simulink model "corrsys"  (R2021a)
settings: Solver=VariableStepAuto  StartTime=0.0  StopTime=0.5  RelTol=1e-3
libraries: slctrlblks x7
settings Model: Creator=Евгений  LastModifiedBy=Евгений

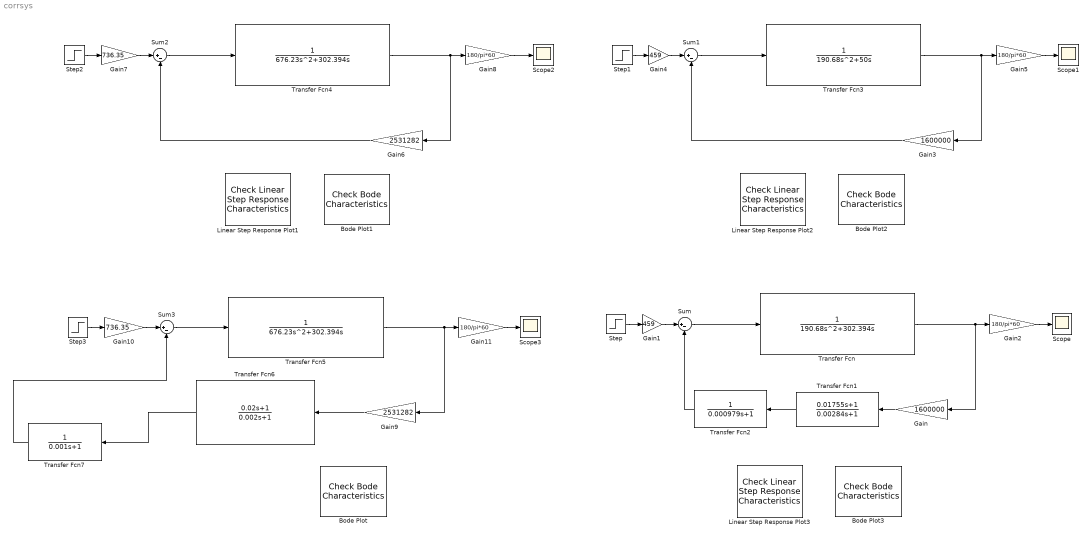
== system corrsys ==
  Bode Plot : slctrlblks/Model Verification/Check Bode  Characteristics  InstantiateOnLoad=on  SaveOperatingPoints=off  LinearizationIOs={'/Gain10', 1, 'in', 'off', '';'/Transfer Fcn7', 1, 'out', 'on', ''}  LinearizeAt=SnapshotTimes  SnapshotTimes=[0]  TriggerType=rising  SampleTime=auto  RateConversionMethod=zoh  PreWarpFreq=10  UseExactDelayModel=off  UseFullBlockNameLabels=off  UseBusSignalLabels=off  enabled=on  stopWhenAssertionFail=off  export=off  ViewDlgPos=[4 4 449 431]  OpenViewOnLoad=off  LaunchViewOnOpen=off  FrequencyUnits=rad/s  MagnitudeUnits=dB  PhaseUnits=deg  TimeUnits=seconds  EnableUpperBound=off  UpperBoundFrequencies=[]  UpperBoundMagnitudes=[]  EnableLowerBound=on  LowerBoundFrequencies=[]  LowerBoundMagnitudes=[]
  Bode Plot1 : slctrlblks/Model Verification/Check Bode  Characteristics  InstantiateOnLoad=on  SaveOperatingPoints=off  LinearizationIOs={'/Gain7', 1, 'in', 'off', '';'/Gain6', 1, 'out', 'on', ''}  LinearizeAt=SnapshotTimes  SnapshotTimes=[0]  TriggerType=rising  SampleTime=auto  RateConversionMethod=zoh  PreWarpFreq=10  UseExactDelayModel=off  UseFullBlockNameLabels=off  UseBusSignalLabels=off  enabled=on  stopWhenAssertionFail=off  export=off  ViewDlgPos=[1 1 1826 895]  OpenViewOnLoad=on  LaunchViewOnOpen=off  FrequencyUnits=rad/s  MagnitudeUnits=dB  PhaseUnits=deg  TimeUnits=seconds  EnableUpperBound=off  UpperBoundFrequencies=[]  UpperBoundMagnitudes=[]  EnableLowerBound=on  LowerBoundFrequencies=[]  LowerBoundMagnitudes=[]
  Bode Plot2 : slctrlblks/Model Verification/Check Bode  Characteristics  InstantiateOnLoad=on  SaveOperatingPoints=off  LinearizationIOs={'/Gain4', 1, 'in', 'off', '';'/Gain3', 1, 'out', 'on', ''}  LinearizeAt=SnapshotTimes  SnapshotTimes=[0]  TriggerType=rising  SampleTime=auto  RateConversionMethod=zoh  PreWarpFreq=10  UseExactDelayModel=off  UseFullBlockNameLabels=off  UseBusSignalLabels=off  enabled=on  stopWhenAssertionFail=off  export=off  ViewDlgPos=[100 200 510 390]  OpenViewOnLoad=off  LaunchViewOnOpen=off  FrequencyUnits=rad/s  MagnitudeUnits=dB  PhaseUnits=deg  TimeUnits=seconds  EnableUpperBound=off  UpperBoundFrequencies=[]  UpperBoundMagnitudes=[]  EnableLowerBound=off  LowerBoundFrequencies=[]  LowerBoundMagnitudes=[]
  Bode Plot3 : slctrlblks/Model Verification/Check Bode  Characteristics  InstantiateOnLoad=on  SaveOperatingPoints=off  LinearizationIOs={'/Gain1', 1, 'in', 'off', '';'/Transfer Fcn2', 1, 'out', 'on', ''}  LinearizeAt=SnapshotTimes  SnapshotTimes=[0]  TriggerType=rising  SampleTime=auto  RateConversionMethod=zoh  PreWarpFreq=10  UseExactDelayModel=off  UseFullBlockNameLabels=off  UseBusSignalLabels=off  enabled=on  stopWhenAssertionFail=off  export=off  ViewDlgPos=[4 5 573 384]  OpenViewOnLoad=off  LaunchViewOnOpen=off  FrequencyUnits=rad/s  MagnitudeUnits=dB  PhaseUnits=deg  TimeUnits=seconds  EnableUpperBound=off  UpperBoundFrequencies=[]  UpperBoundMagnitudes=[]  EnableLowerBound=on  LowerBoundFrequencies=[]  LowerBoundMagnitudes=[]
  Gain : Gain  Gain=1600000
  Gain1 : Gain  Gain=459
  Gain10 : Gain  Gain=736.35
  Gain{2,5,8,11} (4 alike) : Gain  Gain=180/pi*60
  Gain3 : Gain  Gain=1600000
  Gain4 : Gain  Gain=459
  Gain6 : Gain  Gain=2531282
  Gain7 : Gain  Gain=736.35
  Gain9 : Gain  Gain=2531282
  Linear Step Response Plot1 : slctrlblks/Model Verification/Check Linear Step Response Characteristics  InstantiateOnLoad=on  SaveOperatingPoints=off  LinearizationIOs={'/Step2', 1, 'in', 'off', '';'/Gain8', 1, 'out', 'off', ''}  LinearizeAt=SnapshotTimes  SnapshotTimes=[0]  TriggerType=rising  SampleTime=auto  RateConversionMethod=zoh  PreWarpFreq=10  UseExactDelayModel=off  UseFullBlockNameLabels=off  UseBusSignalLabels=off  enabled=on  stopWhenAssertionFail=off  export=off  ViewDlgPos=[1372 4 449 431]  OpenViewOnLoad=off  LaunchViewOnOpen=off  FrequencyUnits=rad/s  MagnitudeUnits=dB  PhaseUnits=deg  TimeUnits=seconds  EnableStepResponseBound=off  FinalValue=[]  RiseTime=[]  PercentRise=[]  SettlingTime=[]  PercentSettling=[]  PercentOvershoot=[]  PercentUndershoot=[]
      settings: SourceProductBaseCode=SD  SaveToWorkspace=off  SaveName=sys
  Linear Step Response Plot2 : slctrlblks/Model Verification/Check Linear Step Response Characteristics  InstantiateOnLoad=on  SaveOperatingPoints=off  LinearizationIOs={'/Step1', 1, 'in', 'off', '';'/Gain5', 1, 'out', 'off', ''}  LinearizeAt=SnapshotTimes  SnapshotTimes=[0]  TriggerType=rising  SampleTime=auto  RateConversionMethod=zoh  PreWarpFreq=10  UseExactDelayModel=off  UseFullBlockNameLabels=off  UseBusSignalLabels=off  enabled=on  stopWhenAssertionFail=off  export=off  ViewDlgPos=[584 417 573 384]  OpenViewOnLoad=off  LaunchViewOnOpen=off  FrequencyUnits=rad/s  MagnitudeUnits=dB  PhaseUnits=deg  TimeUnits=seconds  EnableStepResponseBound=off  FinalValue=[]  RiseTime=[]  PercentRise=[]  SettlingTime=[]  PercentSettling=[]  PercentOvershoot=[]  PercentUndershoot=[]
      settings: SourceProductBaseCode=SD  SaveToWorkspace=off  SaveName=sys
  Linear Step Response Plot3 : slctrlblks/Model Verification/Check Linear Step Response Characteristics  InstantiateOnLoad=on  SaveOperatingPoints=off  LinearizationIOs={'/Step', 1, 'in', 'off', '';'/Gain2', 1, 'out', 'off', ''}  LinearizeAt=SnapshotTimes  SnapshotTimes=[0]  TriggerType=rising  SampleTime=auto  RateConversionMethod=zoh  PreWarpFreq=10  UseExactDelayModel=off  UseFullBlockNameLabels=off  UseBusSignalLabels=off  enabled=on  stopWhenAssertionFail=off  export=off  ViewDlgPos=[584 5 573 384]  OpenViewOnLoad=off  LaunchViewOnOpen=off  FrequencyUnits=rad/s  MagnitudeUnits=dB  PhaseUnits=deg  TimeUnits=seconds  EnableStepResponseBound=off  FinalValue=[]  RiseTime=[]  PercentRise=[]  SettlingTime=[]  PercentSettling=[]  PercentOvershoot=[]  PercentUndershoot=[]
      settings: SourceProductBaseCode=SD  SaveToWorkspace=off  SaveName=sys
  Scope{,1..3} (4 alike) : Scope
  Step{,1..3} (4 alike) : Step  Time=0  SampleTime=0
  Sum{,1..3} (4 alike) : Sum  Inputs=|+-
  Transfer Fcn : TransferFcn  Denominator=[190.68 302.394 0]
  Transfer Fcn1 : TransferFcn  Numerator="[0.01755  1]"  Denominator=[0.00284 1]
  Transfer Fcn2 : TransferFcn  Denominator=[0.000979 1]
  Transfer Fcn3 : TransferFcn  Denominator=[190.68 50 0]
  Transfer Fcn4 : TransferFcn  Denominator=[676.23 302.394 0]
  Transfer Fcn5 : TransferFcn  Denominator=[676.23 302.394 0]
  Transfer Fcn6 : TransferFcn  Numerator=[0.02 1]  Denominator=[0.002 1]
  Transfer Fcn7 : TransferFcn  Denominator="[0.001  1]"
  wires:
  Sum/1 -> Transfer Fcn/1
  Transfer Fcn/1 -> Gain/1, Gain2/1
  Transfer Fcn1/1 -> Transfer Fcn2/1
  Gain/1 -> Transfer Fcn1/1
  Transfer Fcn2/1 -> Sum/2
  Step/1 -> Gain1/1
  Gain1/1 -> Sum/1
  Gain2/1 -> Scope/1
  Transfer Fcn3/1 -> Gain3/1, Gain5/1
  Sum1/1 -> Transfer Fcn3/1
  Step1/1 -> Gain4/1
  Gain4/1 -> Sum1/1
  Gain5/1 -> Scope1/1
  Gain3/1 -> Sum1/2
  Gain6/1 -> Sum2/2
  Sum2/1 -> Transfer Fcn4/1
  Step2/1 -> Gain7/1
  Transfer Fcn4/1 -> Gain6/1, Gain8/1
  Gain7/1 -> Sum2/1
  Gain9/1 -> Transfer Fcn6/1
  Transfer Fcn5/1 -> Gain9/1, Gain11/1
  Sum3/1 -> Transfer Fcn5/1
  Step3/1 -> Gain10/1
  Transfer Fcn6/1 -> Transfer Fcn7/1
  Transfer Fcn7/1 -> Sum3/2
  Gain10/1 -> Sum3/1
  Gain11/1 -> Scope3/1
  Gain8/1 -> Scope2/1
